simulink model "tester"  (R2016b)
settings: Solver=VariableStepAuto  StartTime=0.0  StopTime=10.0  RelTol=1e-3

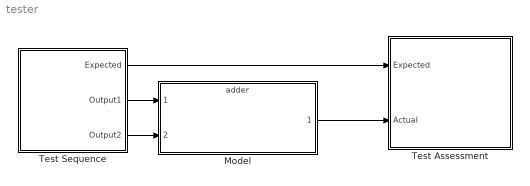
== system tester ==
  Model : ModelReference  ModelNameDialog=adder  SimulationMode=Normal  ModelReferenceVersion=1.2
  Test Assessment : State Transition Table  TreatAsAtomicUnit=on
  Test Sequence : State Transition Table  TreatAsAtomicUnit=on
  wires:
  Test Sequence/1(Expected) -> Test Assessment/1(Expected)
  Test Sequence/3(Output2) -> Model/2
  Test Sequence/2(Output1) -> Model/1
  Model/1 -> Test Assessment/2(Actual)

== stateflow chart tester/Test Assessment ==
  settings: stateMachineType=SIMPLIFIED_MACHINE
  state step_1
    verify(Expected == Actual)
  (default) -> step_1
  data: Expected input; Actual input

== stateflow chart tester/Test Sequence ==
  settings: stateMachineType=SIMPLIFIED_MACHINE
  state step_1
    Output1 = 1;
    Output2 = 1;
    Expected = 2;
  state step_2
    Output1 = 2;
    Output2 = 3;
    Expected = 5;
  (default) -> step_1
  step_1 -> step_2
  data: Expected output; Output1 output; Output2 output
